simulink model "MBD_week1_4"  (R2020b)
settings: Solver=VariableStepAuto  StartTime=0.0  StopTime=10.0  RelTol=1e-3
undefined symbols (not defined in the file): a0, a1, b0, b1
settings Model: Creator=varunraj  LastModifiedBy=varunraj

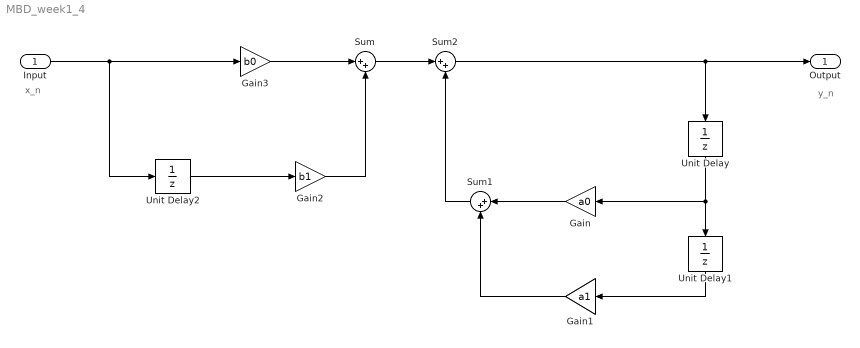
== system MBD_week1_4 ==
  note: y_n
  note: x_n
  Input : Inport
  Gain : Gain  Gain=a0
  Gain1 : Gain  Gain=a1
  Gain2 : Gain  Gain=b1
  Gain3 : Gain  Gain=b0
  Sum : Sum  Inputs=|++
  Sum1 : Sum  Inputs=|++
  Sum2 : Sum  Inputs=|++
  Unit Delay : UnitDelay  SampleTime=-1  HasFrameUpgradeWarning=on
  Unit Delay1 : UnitDelay  SampleTime=-1  HasFrameUpgradeWarning=on
  Unit Delay2 : UnitDelay  SampleTime=-1  HasFrameUpgradeWarning=on
  Output : Outport
  wires:
  Unit Delay/1 -> Gain/1, Unit Delay1/1
  Gain3/1 -> Sum/1
  Unit Delay1/1 -> Gain1/1
  Input/1 -> Unit Delay2/1, Gain3/1
  Sum1/1 -> Sum2/2
  Gain/1 -> Sum1/1
  Sum2/1 -> Unit Delay/1, Output/1
  Gain1/1 -> Sum1/2
  Sum/1 -> Sum2/1
  Unit Delay2/1 -> Gain2/1
  Gain2/1 -> Sum/2
